simulink model "qpsknofilt"  (R2023a)
settings: Solver=ode45  StartTime=0.0  StopTime=0.8e-3  RelTol=1e-3  EnableMultiTasking=on
libraries: commdigbbndpm3 x2, commrandsrc2 x2
CloseFcn:
  | clear qpskSigsOut
Description:
  | Filtered QPSK vs. MSK
  | 
  | This model shows filtered quadrature phase shift keying (QPSK) and minimum shift keying (MSK) modulation schemes and visually compare them.
settings Model: Creator=The MathWorks Inc.  LastModifiedBy=huhan
settings SolverCC: AlgebraicLoopSolver=TrustRegion
settings DataIOCC: SaveFormat=Array  SignalLoggingSaveFormat=ModelDataLogs  SaveOutput=off  SaveTime=off  ReturnWorkspaceOutputs=off  SignalLoggingName=qpskSigsOut
settings OptimizationCC: ExpressionDepthLimit=2147483647  InitFltsAndDblsToZero=on  EfficientMapNaN2IntZero=off  LifeSpan=inf
settings DebuggingCC: SaveWithParameterizedLinksMsg=none  UnderspecifiedInitializationDetection=Classic  MergeDetectMultiDrivingBlocksExec=none  CheckExecutionContextPreStartOutputMsg=on  SignalResolutionControl=TryResolveAllWithWarning  InheritedTsInSrcMsg=none  MultiTaskDSMMsg=warning  MultiTaskCondExecSysMsg=none  SigSpecEnsureSampleTimeMsg=none  FcnCallInpInsideContextMsg=warning  UnconnectedInputMsg=warning  UnconnectedOutputMsg=warning  UnconnectedLineMsg=warning  StateNameClashWarn=warning  SFUnexpectedBacktrackingDiag=warning  SFNoUnconditionalDefaultTransitionDiag=warning  SFExecutionAtInitializationDiag=none  ArithmeticOperatorsInVariantConditions=warning
settings HardwareCC: ProdBitPerPointer=32  ProdBitPerSizeT=32  ProdBitPerPtrDiffT=32  ProdLargestAtomicFloat=None  ProdIntDivRoundTo=Undefined  ProdEndianess=Unspecified  ProdWordSize=32  ProdHWDeviceType=32-bit Generic  TargetUnknown=on
settings ModelReferenceCC: UpdateModelReferenceTargets=IfOutOfDate  PropagateSignalLabelsOutOfModel=off
settings SFSimCC: SimUseLocalCustomCode=off  CustomCodeUndefinedFunction=UseInterfaceOnly
settings RTWCC: RTWUseLocalCustomCode=off
settings CodeAppCC: StateflowObjectComments=on
settings GRTTargetCC: TargetFcnLib=ansi_tfl_tmw.mat  TargetLangStandard=C89/C90 (ANSI)  CombineOutputUpdateFcns=off  GRTInterface=on
settings ConfigComp: CovMetricSettings=dw  CovSaveCumulativeToWorkspaceVar=on  CovSaveSingleToWorkspaceVar=on  CovExternalEMLEnable=off

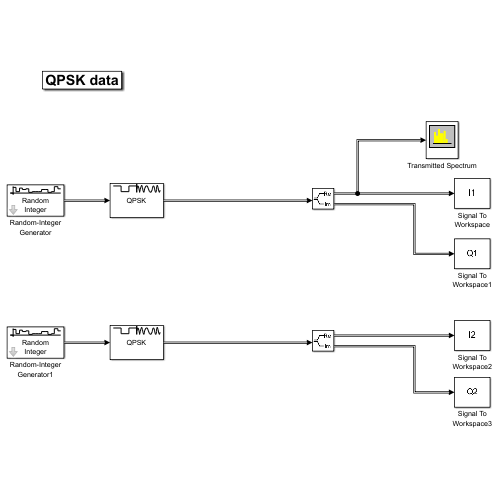
[thumbnail: Simulink's stored preview of the top-level diagram]
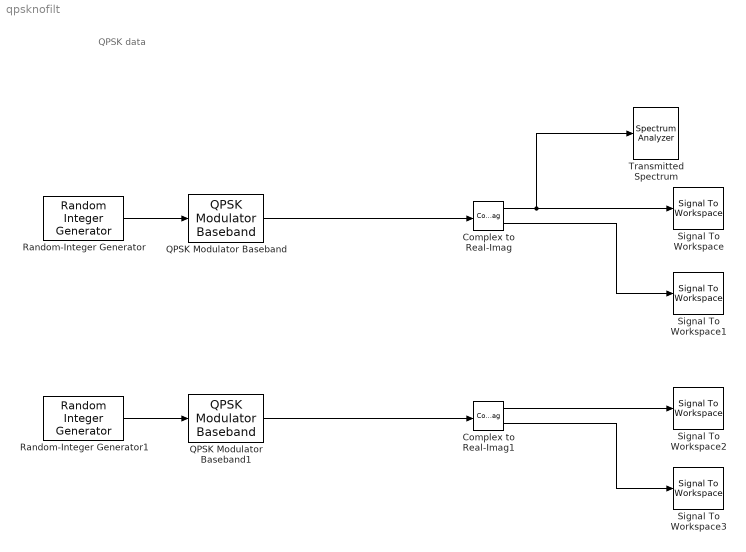
== system qpsknofilt ==
  note: QPSK data
  Complex to Real-Imag : ComplexToRealImag
  Complex to Real-Imag1 : ComplexToRealImag
  QPSK Modulator Baseband : commdigbbndpm3/QPSK Modulator Baseband  InType=Integer  Enc=Binary  Ph=pi/4  outDtype=double  outWordLen=16  outUDDataType=sfix(16)  outFracLenMode=Best precision  outFracLen=15  outDataTypeStr=double  outLastDataTypeStr=double
  QPSK Modulator Baseband1 : commdigbbndpm3/QPSK Modulator Baseband  InType=Integer  Enc=Binary  Ph=pi/4  outDtype=double  outWordLen=16  outUDDataType=sfix(16)  outFracLenMode=Best precision  outFracLen=15  outDataTypeStr=double  outLastDataTypeStr=double
  Random-Integer Generator : commrandsrc2/Random Integer Generator  mul=4  seed=[12345]  Ts=1/(20e6)  frameBased=on  sampPerFrame=100  orient=off  outDataType=int8
  Random-Integer Generator1 : commrandsrc2/Random Integer Generator  mul=4  seed=[12345]  Ts=1/(20e6)  frameBased=on  sampPerFrame=100  orient=off  outDataType=int8
  Signal To Workspace : SignalToWorkspace  VariableName=I1
      settings: CopyFcn=dspblkcopystw(gcbh);
  Signal To Workspace1 : SignalToWorkspace  VariableName=Q1
      settings: CopyFcn=dspblkcopystw(gcbh);
  Signal To Workspace2 : SignalToWorkspace  VariableName=I2
      settings: CopyFcn=dspblkcopystw(gcbh);
  Signal To Workspace3 : SignalToWorkspace  VariableName=Q2
      settings: CopyFcn=dspblkcopystw(gcbh);
  Transmitted Spectrum : SpectrumAnalyzer  WindowPosition=[691.000000,210.000000,800.000000,500.000000,]  ScopeFrameLocation=window  Method=Welch  Span=20000000  StartFrequency=-10000000  StopFrequency=10000000  AveragingMethod=Running  YLimits=[-33.54842383,8.9169021]  DefaultConfigurationName=spbscopes.SpectrumAnalyzerBlockCfg
  wires:
  Complex to Real-Imag/1 -> Transmitted Spectrum/1, Signal To Workspace/1
  Complex to Real-Imag/2 -> Signal To Workspace1/1
  Random-Integer Generator/1 -> QPSK Modulator Baseband/1
  QPSK Modulator Baseband/1 -> Complex to Real-Imag/1
  Complex to Real-Imag1/1 -> Signal To Workspace2/1
  Complex to Real-Imag1/2 -> Signal To Workspace3/1
  Random-Integer Generator1/1 -> QPSK Modulator Baseband1/1
  QPSK Modulator Baseband1/1 -> Complex to Real-Imag1/1
